simulink model "PLL_FOC_Simulation_single"  (R2025b)
settings: Solver=ode3  StartTime=0.0  StopTime=3  FixedStep=Ts/4  RelTol=1e-3
PreLoadFcn:
  | d=fileparts(get_param(bdroot,'FileName'));addpath(d);run(fullfile(d,'obs_params.m'));run(fullfile(d,'foc_ctrl_params.m'))
values from neighbouring files (symbols this model uses):
  a_ho = 2*pi*f_ho_lpf*Ts    [foc_ctrl_params.m]
  f_ho = 25    [foc_ctrl_params.m]
  I_align = 3.0    (= 3)    [foc_ctrl_params.m]
  I_start = 3.0    (= 3)    [foc_ctrl_params.m]
  iq_max = 4    [foc_ctrl_params.m]
  Kp_i = Lc*wc_i    [foc_ctrl_params.m]
  Kp_w = J*wc_w/(p*Kt)    [foc_ctrl_params.m]
  Lc = Ls    [foc_ctrl_params.m]
  psi = 9.2386e-3    (= 0.0092386)    [params_ACT_57BLF02.m]
  t_adc = 1.0    (= 1)    [foc_ctrl_params.m]
  t_align = 0.15    [foc_ctrl_params.m]
  t_ho = t_adc + t_align + t_ramp    (= 1.6)    [foc_ctrl_params.m]
  t_ramp = 0.45    [foc_ctrl_params.m]    (also in obs_params.m = 0.6)
  tau_step = 0.05    [foc_ctrl_params.m]
  tau_step_t = t_adc + 0.7    (= 1.7)    [foc_ctrl_params.m]
  Ts = 1/PWM_frequency    (= 5e-05)    [obs_params.m]    (also in params_ACT_57BLF02.m)
  Tss = 10*Ts    [foc_ctrl_params.m]
  Vmax = Vdc/sqrt(3)    [foc_ctrl_params.m]
  wref = 2*pi*30    (= 188.495559215)    [foc_ctrl_params.m]
undefined symbols (not defined in the file or in its folder): DiscIntNeverNeededParam, pll
libraries: embmathops x1, simulink x1
settings Model: Creator=Lubin Kerhuel  LastModifiedBy=Lubin Kerhuel
settings DataIOCC: ReturnWorkspaceOutputs=off
settings OptimizationCC: LifeSpan=1

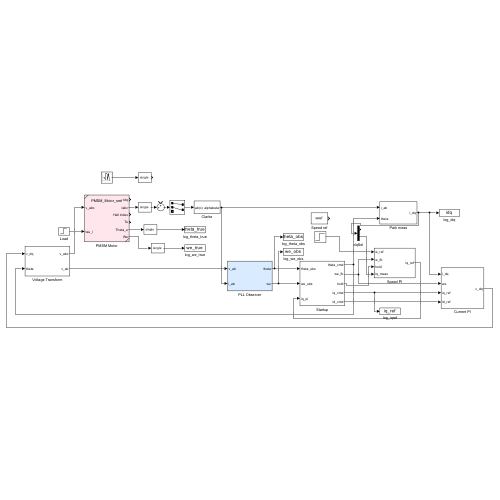
[thumbnail: Simulink's stored preview of the top-level diagram]
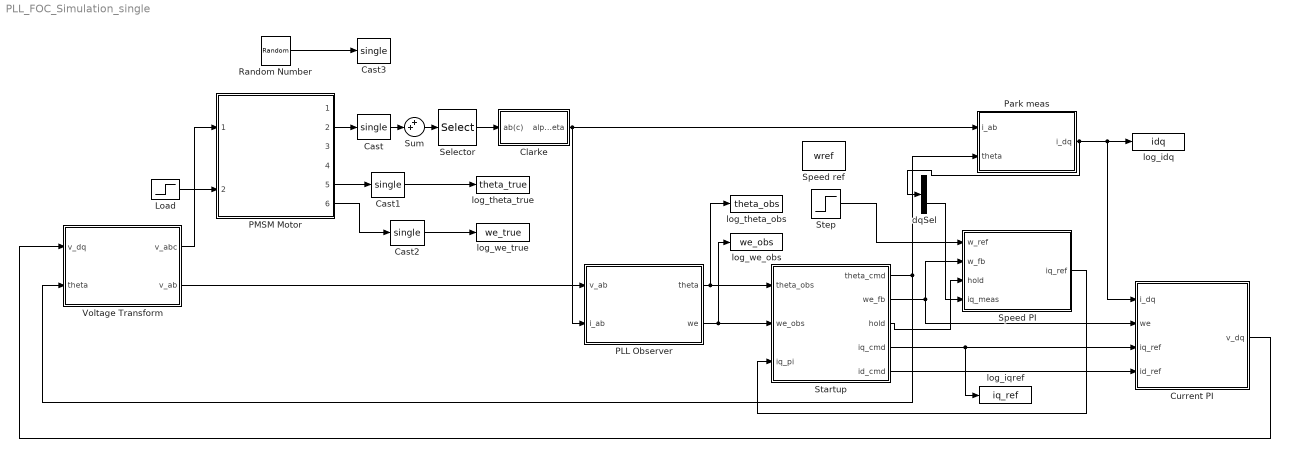
== system PLL_FOC_Simulation_single ==
  Cast{,1..3} (4 alike) : DataTypeConversion  OutDataTypeStr=single  SaturateOnIntegerOverflow=off  RndMeth=Floor
  Clarke : Subsystem
  Current PI : Subsystem
  Load : Step  Time=tau_step_t  After=tau_step  OutDataTypeStr=single  SampleTime=0
  PLL Observer : Subsystem
  PMSM Motor : Subsystem  ReferencedSubsystem=PMSM_Motor_sref
  Park meas : Subsystem
  Random Number : RandomNumber  Variance=0.015  Seed=[22 23 24]  SampleTime=50e-6
  Selector : Selector  InputPortWidth=3  IndexOptions=Index vector (dialog)  Indices=[1 2]  OutputSizes=1
  Speed PI : Subsystem
  Speed ref : Constant  Value=wref  OutDataTypeStr=single
  Startup : Subsystem
  Step : Step  Time=2  Before=180  After=500  OutDataTypeStr=single  SampleTime=Ts
  Sum : Sum  Inputs=++|
  Voltage Transform : Subsystem
  dqSel : Demux  Outputs=2
  log_idq : ToWorkspace  VariableName=idq  SaveFormat=Structure  SampleTime=-1
  log_iqref : ToWorkspace  VariableName=iq_ref  SaveFormat=Timeseries  SampleTime=-1
  log_theta_obs : ToWorkspace  VariableName=theta_obs  SaveFormat=Timeseries  SampleTime=-1
  log_theta_true : ToWorkspace  VariableName=theta_true  SaveFormat=Timeseries  SampleTime=-1
  log_we_obs : ToWorkspace  VariableName=we_obs  SaveFormat=Timeseries  SampleTime=-1
  log_we_true : ToWorkspace  VariableName=we_true  SaveFormat=Timeseries  SampleTime=-1
  wires:
  PMSM Motor/6 -> Cast2/1
  Load/1 -> PMSM Motor/2
  Voltage Transform/1(v_abc) -> PMSM Motor/1
  Voltage Transform/2(v_ab) -> PLL Observer/1(v_ab)
  PLL Observer/1(theta) -> Startup/1(theta_obs), log_theta_obs/1
  PMSM Motor/2 -> Cast/1
  Clarke/1(alphabeta) -> Park meas/1(i_ab), PLL Observer/2(i_ab)
  PMSM Motor/5 -> Cast1/1
  PLL Observer/2(we) -> Startup/2(we_obs), log_we_obs/1
  Park meas/1(i_dq) -> Current PI/1(i_dq), log_idq/1, dqSel/1
  Current PI/1(v_dq) -> Voltage Transform/1(v_dq)
  Selector/1 -> Clarke/1(ab(c))
  Startup/3(hold) -> Speed PI/3(hold)
  Startup/1(theta_cmd) -> Park meas/2(theta), Voltage Transform/2(theta)
  Startup/2(we_fb) -> Speed PI/2(w_fb), Current PI/2(we)
  Speed PI/1(iq_ref) -> Startup/3(iq_pi)
  Step/1 -> Speed PI/1(w_ref)
  Startup/4(iq_cmd) -> log_iqref/1, Current PI/3(iq_ref)
  Startup/5(id_cmd) -> Current PI/4(id_ref)
  Cast/1 -> Sum/2
  Cast1/1 -> log_theta_true/1
  Cast2/1 -> log_we_true/1
  Sum/1 -> Selector/1
  Random Number/1 -> Cast3/1
  dqSel/2 -> Speed PI/4(iq_meas)

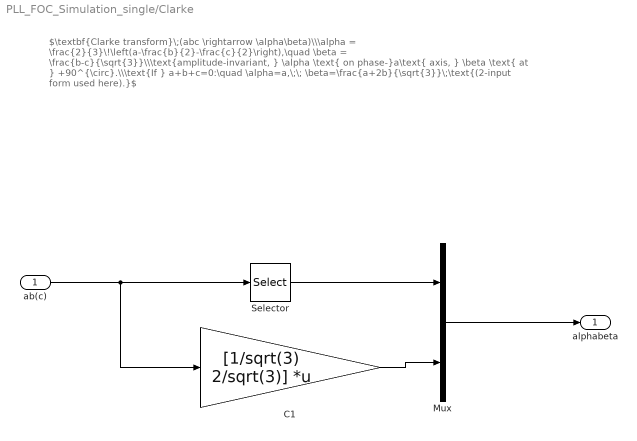
== system PLL_FOC_Simulation_single/Clarke ==
  note: $\textbf{Clarke transform}\;(abc \rightarrow \alpha\beta)\\\alpha = \frac{2}{3}\!\left(a-\frac{b}{2}-\frac{c}{2}\right),\quad \beta = \frac{b-c}{\sqrt{3}}\\\text{amplitude-invariant, } \alpha \text{ on phase-}a\text{ axis, } \beta \text{ at } +90^{\circ}.\\\text{If } a+b+c=0:\quad \alpha=a,\;\; \beta=\frac{a+2b}{\sqrt{3}}\;\text{(2-input form used here).}$
  ab(c) : Inport
  C1 : Gain  Gain=[1/sqrt(3) 2/sqrt(3)]  Multiplication=Matrix(K*u)  OutDataTypeStr=Inherit: Same as input  ParamDataTypeStr=Inherit: Same as input
  Mux : Mux  Inputs=2
  Selector : Selector  InputPortWidth=2  IndexOptions=Index vector (dialog)  Indices=[1]  OutputSizes=1
  alphabeta : Outport  VectorParamsAs1DForOutWhenUnconnected=off
  wires:
  C1/1 -> Mux/2
  Selector/1 -> Mux/1
  Mux/1 -> alphabeta/1
  ab(c)/1 -> C1/1, Selector/1

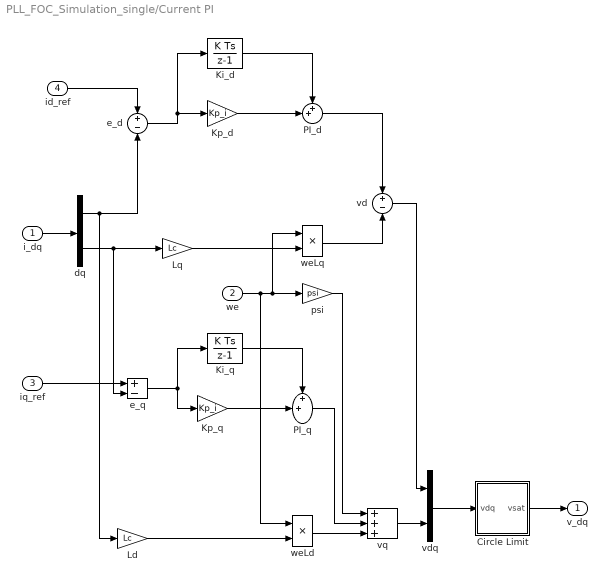
== system PLL_FOC_Simulation_single/Current PI ==
  i_dq : Inport
  we : Inport  Port=2
  iq_ref : Inport  Port=3
  id_ref : Inport  Port=4
  Circle Limit : Subsystem
  Ki_d : DiscreteIntegrator  gainval=Ki_i  SampleTime=Ts  LimitOutput=on  UpperSaturationLimit=Vmax  LowerSaturationLimit=-Vmax  ICPrevOutput=DiscIntNeverNeededParam  ICPrevScaledInput=DiscIntNeverNeededParam
  Ki_q : DiscreteIntegrator  gainval=Ki_i  SampleTime=Ts  LimitOutput=on  UpperSaturationLimit=Vmax  LowerSaturationLimit=-Vmax  ICPrevOutput=DiscIntNeverNeededParam  ICPrevScaledInput=DiscIntNeverNeededParam
  Kp_d : Gain  Gain=Kp_i
  Kp_q : Gain  Gain=Kp_i
  Ld : Gain  Gain=Lc
  Lq : Gain  Gain=Lc
  PI_d : Sum  Inputs=++|
  PI_q : Sum  Inputs=++|
  dq : Demux  Outputs=2
  e_d : Sum  Inputs=+-
  e_q : Sum  Inputs=+-
  psi : Gain  Gain=psi
  vd : Sum  Inputs=+-
  vdq : Mux  Inputs=2
  vq : Sum  Inputs=+++
  weLd : Product  Inputs=**
  weLq : Product  Inputs=**
  v_dq : Outport
  wires:
  i_dq/1 -> dq/1
  dq/2 -> e_q/2, Lq/1
  id_ref/1 -> e_d/1
  iq_ref/1 -> e_q/1
  dq/1 -> e_d/2, Ld/1
  e_q/1 -> Kp_q/1, Ki_q/1
  e_d/1 -> Kp_d/1, Ki_d/1
  Lq/1 -> weLq/2
  Ld/1 -> weLd/2
  weLq/1 -> vd/2
  Ki_d/1 -> PI_d/1
  Kp_d/1 -> PI_d/2
  we/1 -> psi/1, weLq/1, weLd/1
  Ki_q/1 -> PI_q/1
  Kp_q/1 -> PI_q/2
  PI_d/1 -> vd/1
  psi/1 -> vq/1
  PI_q/1 -> vq/2
  Circle Limit/1(vsat) -> v_dq/1
  weLd/1 -> vq/3
  vd/1 -> vdq/1
  vq/1 -> vdq/2
  vdq/1 -> Circle Limit/1(vdq)

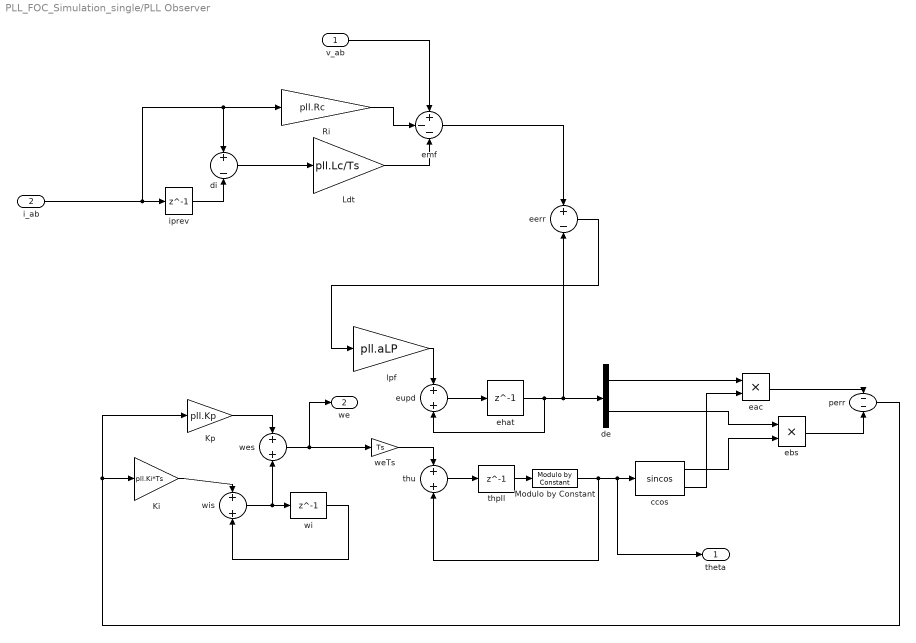
== system PLL_FOC_Simulation_single/PLL Observer ==
  v_ab : Inport
  i_ab : Inport  Port=2
  Ki : Gain  Gain=pll.Ki*Ts
  Kp : Gain  Gain=pll.Kp
  Ldt : Gain  Gain=pll.Lc/Ts
  Modulo by Constant : embmathops/Modulo by Constant  Denominator=2*pi  SimulateUsing=Code generation
      settings: LibrarySourceBlock=embeddedMathLib/Modulo by Constant
  Ri : Gain  Gain=pll.Rc
  ccos : Trigonometry  Operator=sincos
  de : Demux  Outputs=2
  di : Sum  Inputs=+-
  eac : Product  Inputs=**
  ebs : Product  Inputs=**
  eerr : Sum  Inputs=+-
  ehat : Delay  DelayLength=1  InitialCondition=0  SampleTime=Ts
  emf : Sum  Inputs=+--
  eupd : Sum
  iprev : Delay  DelayLength=1  InitialCondition=0  SampleTime=Ts
  lpf : Gain  Gain=pll.aLP
  perr : Sum  Inputs=--
  thpll : Delay  DelayLength=1  InitialCondition=0  SampleTime=Ts
  thu : Sum
  weTs : Gain  Gain=Ts
  wes : Sum
  wi : Delay  DelayLength=1  InitialCondition=0  SampleTime=Ts
  wis : Sum
  theta : Outport  OutDataTypeStr=single
  we : Outport  Port=2  OutDataTypeStr=single
  wires:
  i_ab/1 -> di/1, Ri/1, iprev/1
  wis/1 -> wes/2, wi/1
  iprev/1 -> di/2
  Ri/1 -> emf/2
  wes/1 -> weTs/1, we/1
  di/1 -> Ldt/1
  de/1 -> eac/1
  wi/1 -> wis/2
  lpf/1 -> eupd/1
  ebs/1 -> perr/2
  weTs/1 -> thu/1
  v_ab/1 -> emf/1
  Ldt/1 -> emf/3
  Kp/1 -> wes/1
  eupd/1 -> ehat/1
  thu/1 -> thpll/1
  emf/1 -> eerr/1
  ehat/1 -> de/1, eerr/2, eupd/2
  thpll/1 -> Modulo by Constant/1
  eerr/1 -> lpf/1
  de/2 -> ebs/1
  ccos/2 -> eac/2
  ccos/1 -> ebs/2
  eac/1 -> perr/1
  perr/1 -> Kp/1, Ki/1
  Ki/1 -> wis/1
  Modulo by Constant/1 -> theta/1, ccos/1, thu/2

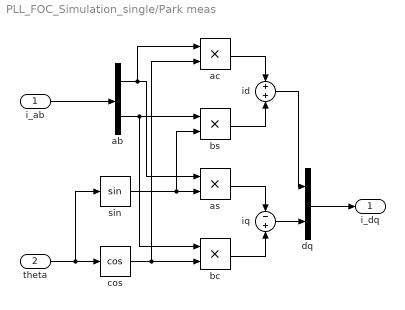
== system PLL_FOC_Simulation_single/Park meas ==
  i_ab : Inport
  theta : Inport  Port=2
  ab : Demux  Outputs=2
  ac : Product  Inputs=**
  as : Product  Inputs=**
  bc : Product  Inputs=**
  bs : Product  Inputs=**
  cos : Trigonometry  Operator=cos
  dq : Mux  Inputs=2
  id : Sum
  iq : Sum  Inputs=-+
  sin : Trigonometry
  i_dq : Outport
  wires:
  i_ab/1 -> ab/1
  sin/1 -> as/2, bs/2
  theta/1 -> cos/1, sin/1
  ab/2 -> bs/1, bc/1
  ab/1 -> ac/1, as/1
  cos/1 -> ac/2, bc/2
  ac/1 -> id/1
  bs/1 -> id/2
  as/1 -> iq/1
  bc/1 -> iq/2
  id/1 -> dq/1
  iq/1 -> dq/2
  dq/1 -> i_dq/1

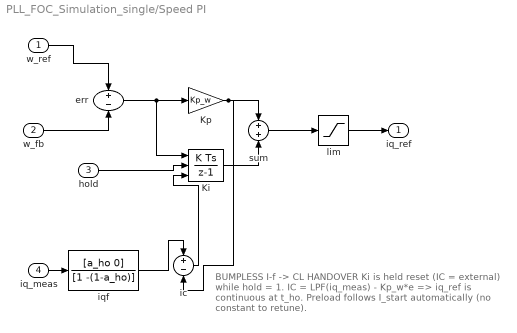
== system PLL_FOC_Simulation_single/Speed PI ==
  note: BUMPLESS I-f -> CL HANDOVER
      | Ki is held reset (IC = external) while hold = 1.
      | IC = LPF(iq_meas) - Kp_w*e  =>  iq_ref is continuous at t_ho.
      | Preload follows I_start automatically (no constant to retune).
  w_ref : Inport
  w_fb : Inport  Port=2
  hold : Inport  Port=3
  iq_meas : Inport  Port=4
  Ki : DiscreteIntegrator  gainval=Ki_w  ExternalReset=level  InitialConditionSource=external  SampleTime=Tss  LimitOutput=on  UpperSaturationLimit=iq_max  LowerSaturationLimit=-iq_max  ICPrevOutput=DiscIntNeverNeededParam  ICPrevScaledInput=DiscIntNeverNeededParam
  Kp : Gain  Gain=Kp_w
  err : Sum  Inputs=+-
  ic : Sum  Inputs=+-
  iqf : DiscreteTransferFcn  Numerator=[a_ho 0]  Denominator=[1 -(1-a_ho)]  SampleTime=Ts
  lim : Saturate  UpperLimit=iq_max  LowerLimit=-iq_max
  sum : Sum
  iq_ref : Outport
  wires:
  w_ref/1 -> err/1
  w_fb/1 -> err/2
  err/1 -> Ki/1, Kp/1
  hold/1 -> Ki/2
  Kp/1 -> sum/1, ic/2
  Ki/1 -> sum/2
  sum/1 -> lim/1
  lim/1 -> iq_ref/1
  iq_meas/1 -> iqf/1
  iqf/1 -> ic/1
  ic/1 -> Ki/3

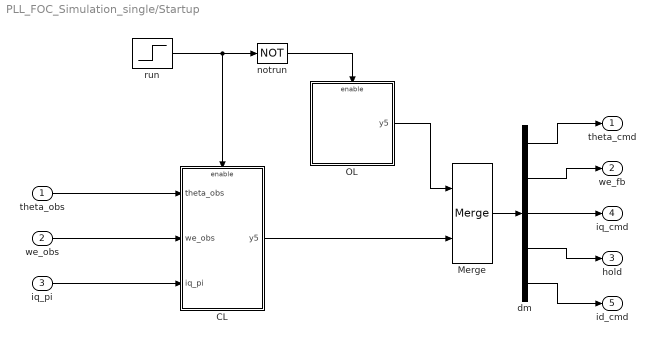
== system PLL_FOC_Simulation_single/Startup ==
  theta_obs : Inport
  we_obs : Inport  Port=2
  iq_pi : Inport  Port=3
  CL : Subsystem  TreatAsAtomicUnit=on
  Merge : Merge
  OL : Subsystem  TreatAsAtomicUnit=on
  dm : Demux  Outputs=5
  notrun : Logic  Operator=NOT  AllPortsSameDT=off  OutDataTypeStr=boolean
  run : Step  Time=t_ho  SampleTime=Ts
  theta_cmd : Outport
  we_fb : Outport  Port=2
  hold : Outport  Port=3
  iq_cmd : Outport  Port=4
  id_cmd : Outport  Port=5
  wires:
  theta_obs/1 -> CL/1(theta_obs)
  notrun/1 -> OL/Enable
  run/1 -> CL/Enable, notrun/1
  dm/1 -> theta_cmd/1
  OL/1(y5) -> Merge/1
  we_obs/1 -> CL/2(we_obs)
  iq_pi/1 -> CL/3(iq_pi)
  CL/1(y5) -> Merge/2
  Merge/1 -> dm/1
  dm/2 -> we_fb/1
  dm/3 -> iq_cmd/1
  dm/4 -> hold/1
  dm/5 -> id_cmd/1

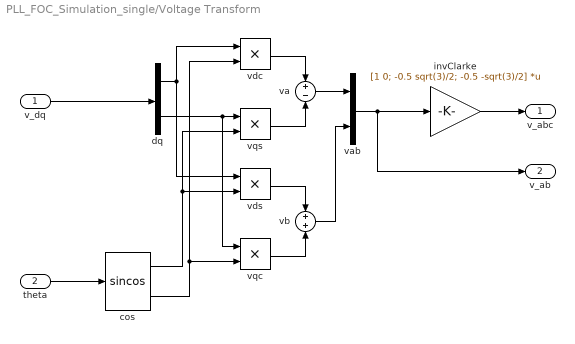
== system PLL_FOC_Simulation_single/Voltage Transform ==
  v_dq : Inport  OutDataTypeStr=single
  theta : Inport  Port=2  OutDataTypeStr=single
  cos : Trigonometry  Operator=sincos
  dq : Demux  Outputs=2
  invClarke : Gain  Gain=[1 0; -0.5 sqrt(3)/2; -0.5 -sqrt(3)/2]  Multiplication=Matrix(K*u)
  va : Sum  Inputs=+-
  vab : Mux  Inputs=2
  vb : Sum
  vdc : Product  Inputs=**
  vds : Product  Inputs=**
  vqc : Product  Inputs=**
  vqs : Product  Inputs=**
  v_abc : Outport
  v_ab : Outport  Port=2
  wires:
  v_dq/1 -> dq/1
  theta/1 -> cos/1
  vqs/1 -> va/2
  cos/1 -> vqs/2, vds/2
  dq/1 -> vdc/1, vds/1
  dq/2 -> vqs/1, vqc/1
  cos/2 -> vdc/2, vqc/2
  invClarke/1 -> v_abc/1
  vdc/1 -> va/1
  vds/1 -> vb/1
  vqc/1 -> vb/2
  va/1 -> vab/1
  vb/1 -> vab/2
  vab/1 -> v_ab/1, invClarke/1

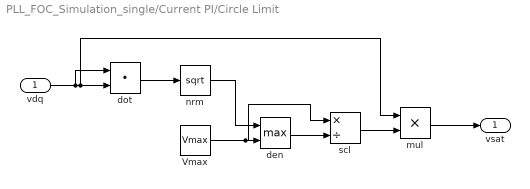
== system PLL_FOC_Simulation_single/Current PI/Circle Limit ==
  vdq : Inport
  Vmax : Constant  Value=Vmax  OutDataTypeStr=single
  den : MinMax  Function=max  Inputs=2
  dot : DotProduct  OutDataTypeStr=Inherit: Inherit via internal rule
  mul : Product  Inputs=**
  nrm : Sqrt
  scl : Product  Inputs=*/
  vsat : Outport
  wires:
  Vmax/1 -> scl/1, den/2
  dot/1 -> nrm/1
  vdq/1 -> mul/1, dot/2, dot/1
  mul/1 -> vsat/1
  nrm/1 -> den/1
  den/1 -> scl/2
  scl/1 -> mul/2

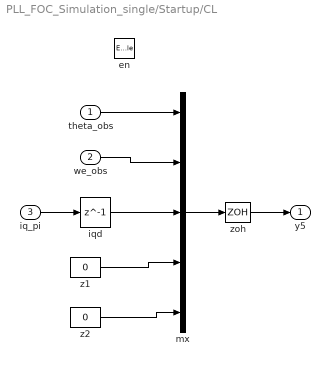
== system PLL_FOC_Simulation_single/Startup/CL ==
  theta_obs : Inport
  we_obs : Inport  Port=2
  iq_pi : Inport  Port=3
  en : EnablePort
  iqd : Delay  DelayLength=1  InitialCondition=0  SampleTime=Ts
  mx : Mux  Inputs=5
  z1 : Constant  Value=0  OutDataTypeStr=single
  z2 : Constant  Value=0  OutDataTypeStr=single
  zoh : ZeroOrderHold  SampleTime=Ts
  y5 : Outport  InitialOutput=[0;0;0;1;0]
  wires:
  iq_pi/1 -> iqd/1
  zoh/1 -> y5/1
  theta_obs/1 -> mx/1
  we_obs/1 -> mx/2
  z1/1 -> mx/4
  iqd/1 -> mx/3
  z2/1 -> mx/5
  mx/1 -> zoh/1

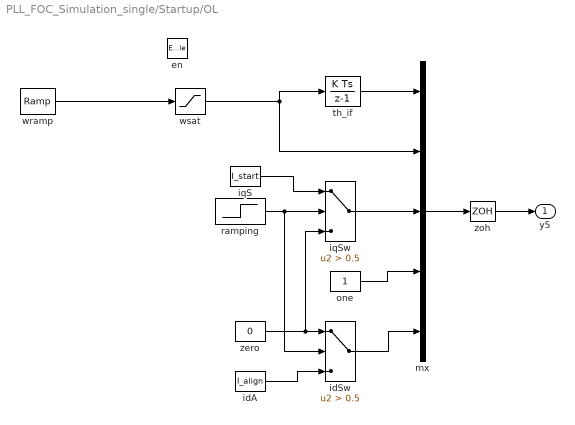
== system PLL_FOC_Simulation_single/Startup/OL ==
  en : EnablePort
  idA : Constant  Value=I_align  OutDataTypeStr=single
  idSw : Switch  Criteria=u2 > Threshold  Threshold=0.5  SaturateOnIntegerOverflow=off  InputSameDT=off
  iqS : Constant  Value=I_start  OutDataTypeStr=single
  iqSw : Switch  Criteria=u2 > Threshold  Threshold=0.5  SaturateOnIntegerOverflow=off  InputSameDT=off
  mx : Mux  Inputs=5
  one : Constant  OutDataTypeStr=single
  ramping : Step  Time=t_adc+t_align  SampleTime=.01
  th_if : DiscreteIntegrator  gainval=1  SampleTime=Ts  ICPrevOutput=DiscIntNeverNeededParam  ICPrevScaledInput=DiscIntNeverNeededParam
  wramp : simulink/Sources/Ramp  slope=2*pi*f_ho/t_ramp  start=t_adc+t_align  InitialOutput=0
  wsat : Saturate  UpperLimit=2*pi*f_ho  LowerLimit=0  OutDataTypeStr=single
  zero : Constant  Value=0  OutDataTypeStr=single
  zoh : ZeroOrderHold  SampleTime=Ts
  y5 : Outport  InitialOutput=[0;0;0;1;0]
  wires:
  wramp/1 -> wsat/1
  zoh/1 -> y5/1
  th_if/1 -> mx/1
  wsat/1 -> mx/2, th_if/1
  idA/1 -> idSw/3
  iqS/1 -> iqSw/1
  iqSw/1 -> mx/3
  ramping/1 -> idSw/2, iqSw/2
  zero/1 -> idSw/1, iqSw/3
  one/1 -> mx/4
  idSw/1 -> mx/5
  mx/1 -> zoh/1
